simulink model "clarke_park_transformations_01"  (R2020b)
settings: Solver=VariableStepAuto  StartTime=0.0  StopTime=0.5  MaxStep=1e-4  RelTol=1e-3
undefined symbols (not defined in the file or in its folder): A_frq_step, A_phase_step, f_rad, t_frq_step, t_phase_step, V_g, var_noise
libraries: simulink x6, bach_library x3
settings Model: Creator=Martin  LastModifiedBy=Martin

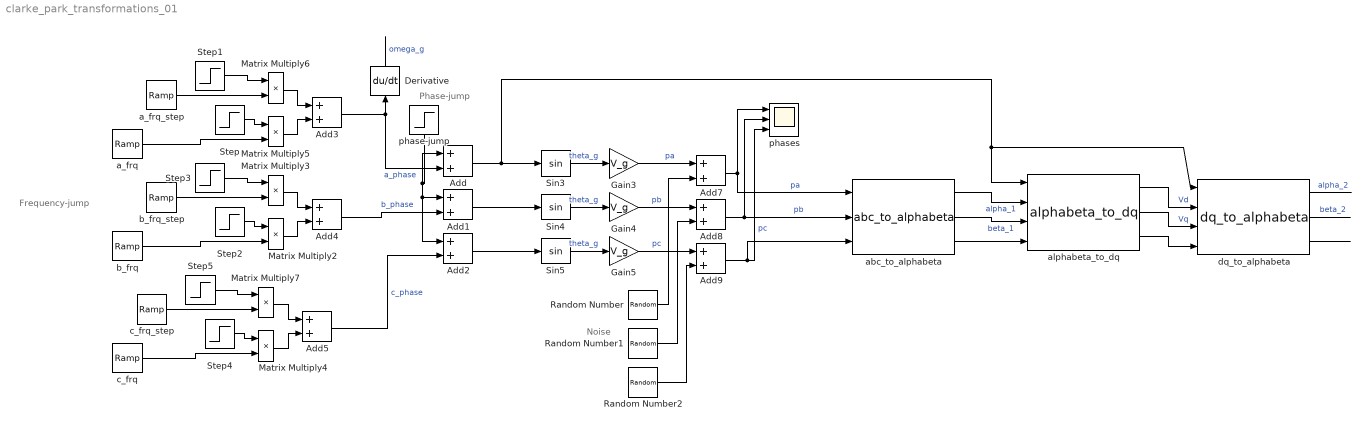
== system clarke_park_transformations_01 ==
  note: Frequency-jump
  note: Phase-jump
  note: Noise
  Add{,1..5,7..9} (9 alike) : Sum
  Derivative : Derivative
  Gain3 : Gain  Gain=V_g
  Gain4 : Gain  Gain=V_g
  Gain5 : Gain  Gain=V_g
  Matrix Multiply{2..7} (6 alike) : Product
  Random Number : RandomNumber  Variance=var_noise
  Random Number1 : RandomNumber  Variance=var_noise  Seed=1
  Random Number2 : RandomNumber  Variance=var_noise  Seed=2
  Sin3 : Trigonometry
  Sin4 : Trigonometry
  Sin5 : Trigonometry
  Step : Step  Time=t_frq_step  Before=1  After=0  SampleTime=0
  Step1 : Step  Time=t_frq_step  SampleTime=0
  Step2 : Step  Time=t_frq_step  Before=1  After=0  SampleTime=0
  Step3 : Step  Time=t_frq_step  SampleTime=0
  Step4 : Step  Time=t_frq_step  Before=1  After=0  SampleTime=0
  Step5 : Step  Time=t_frq_step  SampleTime=0
  a_frq : simulink/Sources/Ramp  slope=f_rad  start=0  InitialOutput=0
  a_frq_step : simulink/Sources/Ramp  slope=f_rad*A_frq_step  start=t_frq_step  InitialOutput=t_frq_step*f_rad
  abc_to_alphabeta : bach_library/abc_to_alphabeta  SystemSampleTime=-1  VariantActivationTime=update diagram  Latency=0  AutoFrameSizeCalculation=off
  alphabeta_to_dq : bach_library/alphabeta_to_dq  SystemSampleTime=-1  VariantActivationTime=update diagram  Latency=0  AutoFrameSizeCalculation=off
  b_frq : simulink/Sources/Ramp  slope=f_rad  start=0  InitialOutput=f_rad/3
  b_frq_step : simulink/Sources/Ramp  slope=f_rad*A_frq_step  start=t_frq_step  InitialOutput=t_frq_step*f_rad+f_rad/3
  c_frq : simulink/Sources/Ramp  slope=f_rad  start=0  InitialOutput=f_rad*2/3
  c_frq_step : simulink/Sources/Ramp  slope=f_rad*A_frq_step  start=t_frq_step  InitialOutput=t_frq_step*f_rad+f_rad*2/3
  dq_to_alphabeta : bach_library/dq_to_alphabeta  SystemSampleTime=-1  VariantActivationTime=update diagram  Latency=0  AutoFrameSizeCalculation=off
  phase-jump : Step  Time=t_phase_step  After=A_phase_step  SampleTime=0
  phases : Scope  NumInputPorts=3
  wires:
  Gain5/1 -> Add9/1  "pc"
  Gain4/1 -> Add8/1  "pb"
  Step5/1 -> Matrix Multiply7/1
  Random Number2/1 -> Add9/2
  b_frq/1 -> Matrix Multiply2/2
  c_frq_step/1 -> Matrix Multiply7/2
  b_frq_step/1 -> Matrix Multiply3/2
  Step3/1 -> Matrix Multiply3/1
  Gain3/1 -> Add7/1  "pa"
  Add/1 -> dq_to_alphabeta/1, alphabeta_to_dq/1, Sin3/1
  Add3/1 -> Add/2, Derivative/1  "a_phase"
  Add9/1 -> abc_to_alphabeta/3, phases/3  "pc"
  Matrix Multiply4/1 -> Add5/2
  Add7/1 -> phases/1, abc_to_alphabeta/1  "pa"
  Add5/1 -> Add2/2  "c_phase"
  Add1/1 -> Sin4/1
  phase-jump/1 -> Add/1, Add2/1, Add1/1
  Random Number/1 -> Add7/2
  c_frq/1 -> Matrix Multiply4/2
  a_frq_step/1 -> Matrix Multiply6/2
  a_frq/1 -> Matrix Multiply5/2
  Sin4/1 -> Gain4/1  "theta_g"
  Matrix Multiply6/1 -> Add3/1
  Matrix Multiply2/1 -> Add4/2
  Sin3/1 -> Gain3/1  "theta_g"
  Add8/1 -> abc_to_alphabeta/2, phases/2  "pb"
  Step4/1 -> Matrix Multiply4/1
  Matrix Multiply7/1 -> Add5/1
  Matrix Multiply3/1 -> Add4/1
  Step/1 -> Matrix Multiply5/1
  Derivative/1 -> ?  "omega_g"
  Add4/1 -> Add1/2  "b_phase"
  Step2/1 -> Matrix Multiply2/1
  Sin5/1 -> Gain5/1  "theta_g"
  Random Number1/1 -> Add8/2
  Step1/1 -> Matrix Multiply6/1
  Add2/1 -> Sin5/1
  Matrix Multiply5/1 -> Add3/2
  abc_to_alphabeta/2 -> alphabeta_to_dq/3  "beta_1"
  abc_to_alphabeta/1 -> alphabeta_to_dq/2  "alpha_1"
  abc_to_alphabeta/3 -> alphabeta_to_dq/4
  alphabeta_to_dq/1 -> dq_to_alphabeta/2  "Vd"
  alphabeta_to_dq/2 -> dq_to_alphabeta/3  "Vq"
  alphabeta_to_dq/3 -> dq_to_alphabeta/4
  dq_to_alphabeta/1 -> ?  "alpha_2"
  dq_to_alphabeta/2 -> ?  "beta_2"
  dq_to_alphabeta/3 -> ?
